simulink model "synchronous_buck_mref"  (R2017b)
settings: Solver=ode1  StartTime=0.0  StopTime=Inf  FixedStep=0.001  RelTol=1e-3
PostLoadFcn:
  | , if any(exist('dsrtsu_mdlpostloadfcn', 'file') == [2, 3, 6]), try dsrtsu_mdlpostloadfcn('Execute', bdroot); catch fprintf('Error in PostLoadFcn (dsrtsu_mdlpostloadfcn) for model "%s":\n %s\n', bdroot, lasterr); end, end,
values from neighbouring files (symbols this model uses):
  C = 500e-6    (= 0.0005)    [init_synchronous_buck_boost.m]
  i_L_init = 1    [init_synchronous_buck_boost.m]
  L = 2e-6    (= 2e-06)    [init_synchronous_buck_boost.m]
  R = 0.5    [init_synchronous_buck_boost.m]
  r_C = 5e-3    (= 0.005)    [init_synchronous_buck_boost.m]
  r_L = 10e-3    (= 0.01)    [init_synchronous_buck_boost.m]
  rds_on_sw1 = 5e-3    (= 0.005)    [init_synchronous_buck_boost.m]
  rds_on_sw2 = 5e-3    (= 0.005)    [init_synchronous_buck_boost.m]
  v_C_init = 3.4    [init_synchronous_buck_boost.m]
Description:
  | Standard RTI1005 template.
  | Supported MATLAB version:  R2017b.
settings Model: Tag=RTI1005  DSRTSU_INTERNAL_RTI_VER=540  DSRTSU_INTERNAL_RTI_TYPE=rti1005  RTICANMMDATA=struct('GeneralSetupData',struct('modelroot','C:\Projects\Simulink\PE_1\w2','generalsettings',struct('filesettings',struct('destfolder',struct('Name','RTICANMM_FILES','Check',1),'buildfolder',struct('Name','.','Check',1),'AbsDestfolder',struct('Name','C:\Projects\Simulink\PE_1\w2\RTICANMM_FILES'),'AbsBuildfolder',struct('Name','C:\Projects\Simulink\PE_1\w2'))),'options',struct('addpaths',1,'rmpaths',1,'addtrcexclusion',logical(1),'cannavigator',struct('checkmonitoring',0),'show_usrtrc',0,'use_usrtrc',0),'advanced',struct('options',ones(1,100)),'MPSetup',{{}},'RTI',struct('Type','RTI1005','Ver','7.12','Date','02-May-2019'),'modelname','synchronous_buck_mref','block','synchronous_buck_mref'))  DSRTSU_INTERNAL_RTIFPGA=130  Creator=CA72672  LastModifiedBy=CA72672
settings OptimizationCC: BlockReduction=off  OptimizeBlockIOStorage=off  BufferReuse=off  GlobalBufferReuse=off  ExpressionFolding=off  LocalBlockOutputs=off
settings HardwareCC: ProdBitPerPointer=32  ProdBitPerSizeT=32  ProdBitPerPtrDiffT=32  ProdLargestAtomicInteger=Integer  ProdEndianess=BigEndian  ProdWordSize=32  ProdHWDeviceType=Custom Processor->Custom  TargetIntDivRoundTo=Zero  TargetEndianess=BigEndian  TargetHWDeviceType=Custom Processor->Custom
settings SFSimCC: MATLABDynamicMemAlloc=off
settings RTWCC: SystemTargetFile=rti1005.tlc  MakeCommand=make_rti  TemplateMakefile=rti1005.tmf  Description=dSPACE DS1005 Hardware Platform
settings CodeAppCC: StateflowObjectComments=on
settings STFCustomTargetCC: ParMdlRefBuildCompliant=on  MatFileLogging=on  GRTInterface=off  SystemTargetFile=rti1005.tlc
settings GRTTargetCC: TargetLangStandard=C89/C90 (ANSI)  CompOptLevelCompliant=off  ConcurrentExecutionCompliant=off  CombineOutputUpdateFcns=off  CPPClassGenCompliant=off  UseToolchainInfoCompliant=off
settings ConfigComp: CovMetricSettings=dswe

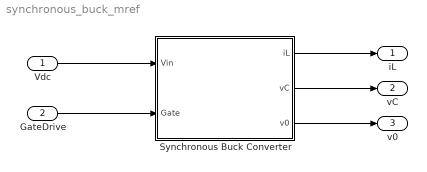
== system synchronous_buck_mref ==
  Vdc : Inport
  GateDrive : Inport  Port=2
  Synchronous Buck Converter : Subsystem
  iL : Outport
  vC : Outport  Port=2
  v0 : Outport  Port=3
  wires:
  Vdc/1 -> Synchronous Buck Converter/1(Vin)
  GateDrive/1 -> Synchronous Buck Converter/2(Gate)
  Synchronous Buck Converter/1(iL) -> iL/1
  Synchronous Buck Converter/2(vC) -> vC/1
  Synchronous Buck Converter/3(v0) -> v0/1

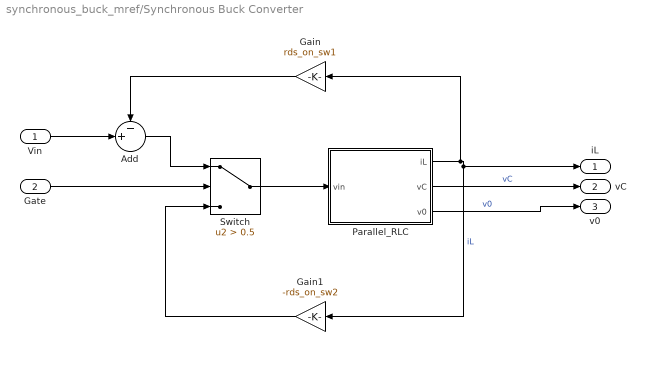
== system synchronous_buck_mref/Synchronous Buck Converter ==
  Vin : Inport
  Gate : Inport  Port=2
  Add : Sum  Inputs=-+|
  Gain : Gain  Gain=rds_on_sw1
  Gain1 : Gain  Gain=-rds_on_sw2
  Parallel_RLC : Subsystem
  Switch : Switch  Criteria=u2 > Threshold  Threshold=0.5
  iL : Outport
  vC : Outport  Port=2
  v0 : Outport  Port=3
  wires:
  Switch/1 -> Parallel_RLC/1(vin)
  Gain1/1 -> Switch/3
  Gain/1 -> Add/1
  Parallel_RLC/2(vC) -> vC/1  "vC"
  Parallel_RLC/1(iL) -> Gain1/1, iL/1, Gain/1  "iL"
  Add/1 -> Switch/1
  Parallel_RLC/3(v0) -> v0/1  "v0"
  Vin/1 -> Add/2
  Gate/1 -> Switch/2

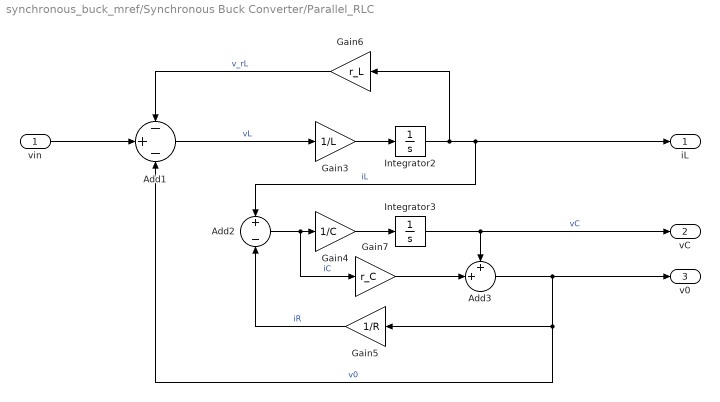
== system synchronous_buck_mref/Synchronous Buck Converter/Parallel_RLC ==
  vin : Inport
  Add1 : Sum  Inputs=-+-
  Add2 : Sum  Inputs=+|-
  Add3 : Sum  Inputs=++|
  Gain3 : Gain  Gain=1/L
  Gain4 : Gain  Gain=1/C
  Gain5 : Gain  Gain=1/R
  Gain6 : Gain  Gain=r_L
  Gain7 : Gain  Gain=r_C
  Integrator2 : Integrator  InitialCondition=i_L_init
  Integrator3 : Integrator  InitialCondition=v_C_init
  iL : Outport
  vC : Outport  Port=2
  v0 : Outport  Port=3
  wires:
  Add3/1 -> Gain5/1, Add1/3, v0/1  "v0"
  Gain7/1 -> Add3/2
  Gain6/1 -> Add1/1  "v_rL"
  Integrator3/1 -> Add3/1, vC/1  "vC"
  Gain5/1 -> Add2/2  "iR"
  Add2/1 -> Gain4/1, Gain7/1  "iC"
  Gain4/1 -> Integrator3/1
  Integrator2/1 -> iL/1, Add2/1, Gain6/1  "iL"
  Gain3/1 -> Integrator2/1
  Add1/1 -> Gain3/1  "vL"
  vin/1 -> Add1/2
